simulink model "stream_in_stream_out"  (R2019b)
settings: Solver=VariableStepAuto  StartTime=0.0  StopTime=9  RelTol=1e-3
undefined symbols (not defined in the file): xc7vx485tffg1157
libraries: ModelComposer x5
settings Model: Creator=viswanad  LastModifiedBy=abehbood
settings DataIOCC: ReturnWorkspaceOutputs=off
settings SFSimCC: CustomCodeUndefinedFunction=UseInterfaceOnly

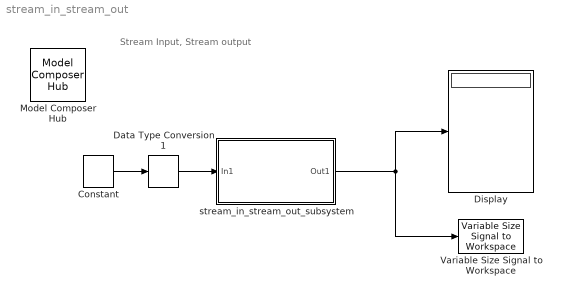
== system stream_in_stream_out ==
  note: Stream Input, Stream output
  Constant : ModelComposer/Constant  Value=[1 2 3 4 5 6 7 8]  SampleTime=1  OutDataType=double  TypeExp=''  Signedness=Signed  WordLength=16  FractionalLength=0  RoundingMode=Truncation to minus infinity  OverflowMode=Wrap around
  Data Type Conversion1 : ModelComposer/Data Type Conversion  OutDataType=int32  TypeExp=''  Signedness=Signed  WordLength=16  FractionalLength=0  RoundingMode=Truncation to minus infinity  OverflowMode=Wrap around
  Display : Display
  Model Composer Hub : ModelComposer/Model Composer Hub  CodeGeneration=off  SubsystemName=stream_in_stream_out_subsystem  TargetDirectory=./code  ExportType=AI Engines  IpVendor=xilinx.com  IpLibrary=hls  IpVersion=1.0  IpHWLanguage=Verilog  AieCompilerOptions={}  CreateTestbench=on  TestbenchStackSize=10  RunAieSim=on  AieSimTimeout=50000  LaunchVitisAnalyzer=off  RunX86Sim=off  X86SimTimeout=10  ProjDevice=xc7vx485tffg1157-1  ProjDevicePart=xc7vx485tffg1157-1  SamplePeriod=-1  ClockFrequency=200  DataPathParallelism=1
  Variable Size Signal to Workspace : ModelComposer/Variable Size Signal to Workspace  VariableNameMask=simout
  stream_in_stream_out_subsystem : Subsystem
  wires:
  Constant/1 -> Data Type Conversion1/1
  stream_in_stream_out_subsystem/1(Out1) -> Variable Size Signal to Workspace/1, Display/1
  Data Type Conversion1/1 -> stream_in_stream_out_subsystem/1(In1)

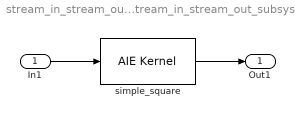
== system stream_in_stream_out/stream_in_stream_out_subsystem ==
  In1 : Inport
  simple_square : ModelComposer/AIE Kernel  PortAttributesTable={ 'Input', 'in', 'input_stream_int32 *', '', '', '', ''; 'Output', 'out', 'output_stream_int32 *', '', '', '', '16' }  PortAttributesEnablement={'off', 'off', 'off', 'off', 'off', 'off', 'off';'off', 'off', 'off', 'off', 'off', 'off', 'on'}  FormalArgDecls={'input_stream_int32 * in', 'output_stream_int32 * out'}  PortWindowSizes={0.000000000000000000e+00, 0.000000000000000000e+00}  PortWindowMargins={0.000000000000000000e+00, 0.000000000000000000e+00}  PortSynchronicities={'auto', 'auto'}  PortSignalSizes={0.000000000000000000e+00, 1.600000000000000000e+01}  SimLibPath=''  FunctionTabVisible=on  FunctionDescription=void simple_square(input_stream_int32 * in, output_stream_int32 * out)  KernelHeaderFile=src/kernels/stream_in_stream_out.h  KernelFunction=simple_square  KernelFunctionSelect=<empty>  KernelSourceFile=src/kernels/stream_in_stream_out.cc  KernelSearchPaths={}  PreProcOptions={}  CoreRuntimeRatio=0.9
  Out1 : Outport  VectorParamsAs1DForOutWhenUnconnected=off
  wires:
  In1/1 -> simple_square/1
  simple_square/1 -> Out1/1
